simulink model "MatchedFilterFFT_Transpose"  (R2021a)
settings: Solver=FixedStepDiscrete  StartTime=0.0  StopTime=inf  RelTol=1e-3
InitFcn:
  | FFT2D_matrix_init
values from neighbouring files (symbols this model uses):
  columnWindowFun = taylorwin(nCols,10,-40)    [FFT2D_matrix_init.m]
  DTsig_in = numerictype(1,20,18)    [FFT2D_matrix_init.m]
  DTWindowFun = numerictype(1,16+4,13+4)    [FFT2D_matrix_init.m]
  nCols = 64    [FFT2D_matrix_init.m]
  nRows = 256    [FFT2D_matrix_init.m]
  radarDataCube = createRadarDataCubeMod(     txSignalFullPeriod,antennaElement,Fs,Fc,      targetPos, targetVel, targetRCS,      RngMax, RxActiveTime, RngGate,      CPILength, NumCPI, CPILength*pulsePeriod)    [FFT2D_matrix_init.m]
libraries: hdlsllib x35, simulink x13, hwlogicconnlib x2, dsphdlfiltering x1, dsphdlxfrm x1, dspsrcs4 x1
(part 1 of 2)
Description:
  | GenericDesign_AX4Master
  | 
  | Template model for GenericDesign ADC/DAC inports/outports with master/slave DMA connection and AXI4 Master
settings Model: DataTypeOverride=Off  SimulationMode=accelerator  Creator=darenlee  LastModifiedBy=darenlee
settings SolverCC: AlgebraicLoopSolver=TrustRegion
settings DataIOCC: SaveOutput=off  SaveTime=off
settings OptimizationCC: BlockReduction=off  ConditionallyExecuteInputs=off  DefaultParameterBehavior=Inlined
settings DebuggingCC: AlgebraicLoopMsg=error  SingleTaskRateTransMsg=error  SFMachineParentedDataDiag=warning
settings HardwareCC: ProdBitPerPointer=32  ProdBitPerSizeT=32  ProdBitPerPtrDiffT=32  ProdLargestAtomicFloat=None  ProdIntDivRoundTo=Undefined  ProdEndianess=Unspecified  ProdWordSize=32  ProdHWDeviceType=ASIC/FPGA->ASIC/FPGA  TargetBitPerPointer=64  TargetBitPerSizeT=64  TargetBitPerPtrDiffT=64  TargetLongLongMode=on  TargetIntDivRoundTo=Zero  TargetEndianess=LittleEndian  TargetWordSize=64  TargetHWDeviceType=Custom Processor->MATLAB Host Computer  ProdEqTarget=off
settings SFSimCC: CustomCodeUndefinedFunction=UseInterfaceOnly

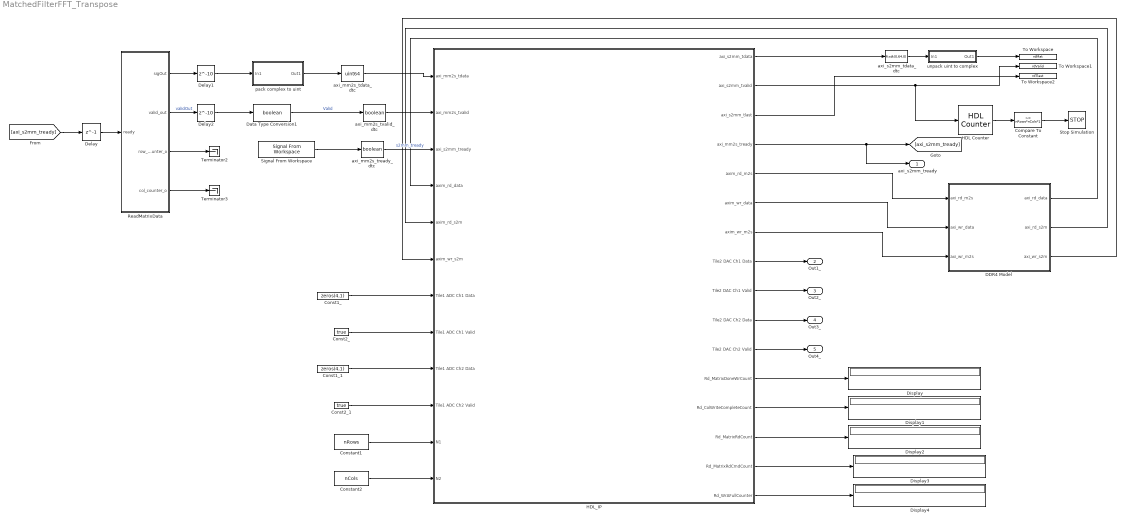
== system MatchedFilterFFT_Transpose ==
  Compare To Constant : simulink/Logic and Bit Operations/Compare To Constant  relop=>=  const=nRows*nCols*1  OutDataTypeStr=boolean
  Const1_ : Constant  Value=zeros(4,1)  OutDataTypeStr=uint64  SampleTime=-1
  Const1_1 : Constant  Value=zeros(4,1)  OutDataTypeStr=uint64  SampleTime=-1
  Const2_ : Constant  Value=true  OutDataTypeStr=boolean  SampleTime=-1
  Const2_1 : Constant  Value=true  OutDataTypeStr=boolean  SampleTime=-1
  Constant1 : Constant  Value=nRows  OutDataTypeStr=uint32  SampleTime=-1
  Constant2 : Constant  Value=nCols  OutDataTypeStr=uint32  SampleTime=-1
  DDR4 Model : Subsystem
  Data Type Conversion1 : DataTypeConversion  OutDataTypeStr=boolean
  Delay : Delay  DelayLength=1
  Delay1 : Delay  DelayLength=10
  Delay2 : Delay  DelayLength=10
  Display{,1..4} (5 alike) : Display
  HDL Counter : hdlsllib/Sources/HDL Counter  CountType=Free running  CountInit=0  CountStep=1  CountMax=25  CountFromType=Initial value  CountFrom=0  CountResetPort=off  CountLoadPort=off  CountEnbPort=on  CountDirPort=off  CountHitOutputPort=off  CountDataType=Unsigned  CountWordLen=32  CountFracLen=0  CountSampTime=1
  HDL_IP : Subsystem  TreatAsAtomicUnit=on
  ReadMatrixData : MATLAB Function  TreatAsAtomicUnit=on  SystemSampleTime=Ts  mask{MatrixInput=radarDataCube, ValidGap=512*3 % 48 clock cycles, Ts=1}
      mask prompts: MatrixInput "Matrix value"; ValidGap "Valid Gap between columns"; Ts "Sample Time"
  Signal From Workspace : dspsrcs4/Signal From Workspace  X=true  Ts=1  nsamps=1  OutputAfterFinalValue=Cyclic repetition  ignoreOrWarnInputAndFrameLengths=off  OutputFrames=off
  Stop Simulation : Stop
  Terminator2 : Terminator
  Terminator3 : Terminator
  To Workspace : ToWorkspace  VariableName=rdMat  SampleTime=-1
      settings: Save2DSignal=2-D array (concatenate along first dimension)
  To Workspace1 : ToWorkspace  VariableName=rdValid  SampleTime=-1
      settings: Save2DSignal=2-D array (concatenate along first dimension)
  To Workspace2 : ToWorkspace  VariableName=rdTlast  SampleTime=-1
      settings: Save2DSignal=2-D array (concatenate along first dimension)
  axi_mm2s_tdata_dtc : DataTypeConversion  OutDataTypeStr=uint64  ConvertRealWorld=Stored Integer (SI)
  axi_mm2s_tready_dtc : DataTypeConversion  OutDataTypeStr=boolean
  axi_mm2s_tvalid_dtc : DataTypeConversion  OutDataTypeStr=boolean
  axi_s2mm_tdata_dtc : DataTypeConversion  OutDataTypeStr=fixdt(0,64,0)  ConvertRealWorld=Stored Integer (SI)
  pack complex to uint : Subsystem
  "unpack uint to complex " : Subsystem
  axi_s2mm_tready : Outport  VectorParamsAs1DForOutWhenUnconnected=off
  Out1_ : Outport  Port=2
  Out2_ : Outport  Port=3
  Out3_ : Outport  Port=4
  Out4_ : Outport  Port=5
  wires:
  HDL_IP/11(Tile2 DAC Ch2 Valid) -> Out4_/1
  axi_mm2s_tvalid_dtc/1 -> HDL_IP/2(axi_mm2s_tvalid)
  Const2_1/1 -> HDL_IP/10(Tile1 ADC Ch2 Valid)
  Const1_1/1 -> HDL_IP/9(Tile1 ADC Ch2 Data)
  HDL_IP/10(Tile2 DAC Ch2 Data) -> Out3_/1
  DDR4 Model/3("axi_wr_s2m ") -> HDL_IP/6(axim_wr_s2m)
  Const2_/1 -> HDL_IP/8(Tile1 ADC Ch1 Valid)
  Const1_/1 -> HDL_IP/7(Tile1 ADC Ch1 Data)
  HDL_IP/9(Tile2 DAC Ch1 Valid) -> Out2_/1
  HDL_IP/8(Tile2 DAC Ch1 Data) -> Out1_/1
  DDR4 Model/1(axi_rd_data) -> HDL_IP/4(axim_rd_data)
  DDR4 Model/2("axi_rd_s2m ") -> HDL_IP/5(axim_rd_s2m)
  HDL_IP/7(axim_wr_m2s) -> DDR4 Model/3(axi_wr_m2s)
  HDL_IP/6(axim_wr_data) -> DDR4 Model/2(axi_wr_data)
  HDL_IP/5(axim_rd_m2s) -> DDR4 Model/1(axi_rd_m2s)
  Signal From Workspace/1 -> axi_mm2s_tready_dtc/1
  Data Type Conversion1/1 -> axi_mm2s_tvalid_dtc/1  "Valid"
  HDL_IP/1(axi_s2mm_tdata) -> axi_s2mm_tdata_dtc/1
  axi_mm2s_tdata_dtc/1 -> HDL_IP/1(axi_mm2s_tdata)
  HDL_IP/4(axi_mm2s_tready) -> axi_s2mm_tready/1, [axi_s2mm_tready]
  axi_mm2s_tready_dtc/1 -> HDL_IP/3(axi_s2mm_tready)  "s2mm_tready"
  ReadMatrixData/4(col_counter_o) -> Terminator3/1
  ReadMatrixData/3(row_counter_o) -> Terminator2/1
  ReadMatrixData/2(valid_out) -> Delay2/1  "validOut"
  ReadMatrixData/1(sigOut) -> Delay1/1
  Compare To Constant/1 -> Stop Simulation/1
  HDL_IP/2(axi_s2mm_tvalid) -> To Workspace1/1, HDL Counter/1
  HDL Counter/1 -> Compare To Constant/1
  axi_s2mm_tdata_dtc/1 -> "unpack uint to complex "/1(In1)
  [axi_s2mm_tready] -> Delay/1
  Delay/1 -> ReadMatrixData/1(ready)
  Constant1/1 -> HDL_IP/11(N1)
  Constant2/1 -> HDL_IP/12(N2)
  Delay2/1 -> Data Type Conversion1/1
  HDL_IP/12(Rd_MatrixDoneWrCount) -> Display/1
  HDL_IP/13(Rd_ColWriteCompleteCount) -> Display1/1
  HDL_IP/14(Rd_MatrixRdCount) -> Display2/1
  HDL_IP/15(Rd_MatrixRdCmdCount) -> Display3/1
  HDL_IP/16(Rd_WrAFullCounter) -> Display4/1
  HDL_IP/3(axi_s2mm_tlast) -> To Workspace2/1
  Delay1/1 -> pack complex to uint/1(In1)
  pack complex to uint/1(Out1) -> axi_mm2s_tdata_dtc/1
  "unpack uint to complex "/1(Out1) -> To Workspace/1

== system MatchedFilterFFT_Transpose/DDR4 Model ==
  axi_rd_m2s : Inport
  axi_wr_data : Inport  Port=2
  axi_wr_m2s : Inport  Port=3
  DDR1 : Subsystem  mask{DDR3_DEPTH=1024, WR_RD_DATAWIDTH=64, INIT_DDR3=off, INIT_ADDR=0, INIT_DATA=fi(zeros(1,1024),0,64,0), OutDataTypeStr=fixdt(0,64,0), READY_DUTY_CYL=1, toggle=off}
      mask prompts: DDR3_DEPTH "DDR DEPTH"; WR_RD_DATAWIDTH "DDR Data Width"; INIT_DDR3 "Initialize DDR"; INIT_ADDR "DDR Initial Address"; INIT_DATA "DDR Initialization data"; OutDataTypeStr "Simulink:blkprm_prompts:UNIFIEDDATATYPE"; READY_DUTY_CYL "READY Duty Cycle"; toggle "Read Valid Toggling"
      mask help: DDR Simulation model
      mask init:
      | if(DDR3_DEPTH<=1)
      |     error('DDR size should be greater than 1' )  
      | end
      | 
      | if(READY_DUTY_CYL>1)
      |   error('should be less than 1' )  
      | end
      |    
      | 
      | %%Initialization Value
      | if(INIT_DDR3==true)
      |     if(isempty(INIT_ADDR))
      |      error('Enter Initial address' )  
      |     end   
      | end
      | 
      | % Check bit-width
      | checkBitdepth = log2(WR_RD_DATAWIDTH);
      | if floor(checkBitdepth) ~= ceil(checkBitdepth)
      |     error('Bit width is not of power base 2!')
      | end
      | 
      | % Check that bit-width matches the initialization data
      | if INIT_DDR3
      |     init_dt_wl = OutDataTypeStr.WordLength;
      |     init_data_wl = INIT_DATA.WordLength;
      |     if init_dt_wl ~= WR_RD_DATAWIDTH
      |         error('Initialization data type and DDR data width should match!')
      |     end
      |     
      |     if init_data_wl ~= WR_RD_DATAWIDTH
      |         error('Initialization data must match DDR data width!')
      |     end    
      | end
      | 
      | 
      | DT_OUTPUT_TYPE = fixdt(0,WR_RD_DATAWIDTH,0);
      mask Help: DDR Simulation model
      mask TypeOptions WR_RD_DATAWIDTH: 32 | 64 | 128
      mask Callback INIT_DDR3:
      | % Get the mask parameter values. This is a cell
      | %   array of character vectors.
      | maskStr = get_param(gcb,'INIT_DDR3');
      | 
      | % The pop-up menu is the first mask parameter.
      | %   Check the value selected in the pop-up
      | if strcmp(maskStr,'on')
      | 
      |     % Set the visibility of both parameters on when
      |     %   User-defined is selected in the pop-up.
      | 
      |     set_param(gcb,'MaskEnables',{'on','on','on','on','on','on','on','on'});
      | 
      | else
      | 
      |     % Turn off the visibility of the Value field
      |     %   when User-defined is not selected.
      | 
      |     set_param(gcb,'MaskEnables',{'on','on','on','off','off','on','on','on'});
      | 
      |     % Set the character vector in the Values field equal to the
      |     % character vector selected in the Gain pop-up menu.
      | 
      |     %maskStr{2}=maskStr{1};
      | 
      | end
      mask TypeOptions OutDataTypeStr: axi_wr_data/OutDataTypeStr | axi_rd_data/OutDataTypeStr
      mask DialogControl DescGroupVar Prompt: DDR
      mask DialogControl DDR3_INIT Prompt: DDR Initialization
      mask DialogControl PARAM_GROUP Prompt: DDR Initialization Parameters
      mask DialogControl OutDataTypeStr Prompt: Data type:
      mask DialogControl READY_DUTY_CYL Tooltip: between 0 to 1
  Terminator : Terminator
  axi_rd_data : Outport
  "axi_rd_s2m " : Outport  Port=2
  "axi_wr_s2m " : Outport  Port=3
  wires:
  axi_rd_m2s/1 -> DDR1/1(axi_rd_m2s)
  axi_wr_data/1 -> DDR1/2(axi_wr_data)
  axi_wr_m2s/1 -> DDR1/3(axi_wr_m2s)
  DDR1/2(axi_rd_data) -> axi_rd_data/1
  DDR1/3(axi_rd_s2m) -> "axi_rd_s2m "/1
  DDR1/4(axi_wr_s2m) -> "axi_wr_s2m "/1
  DDR1/1(load_done) -> Terminator/1

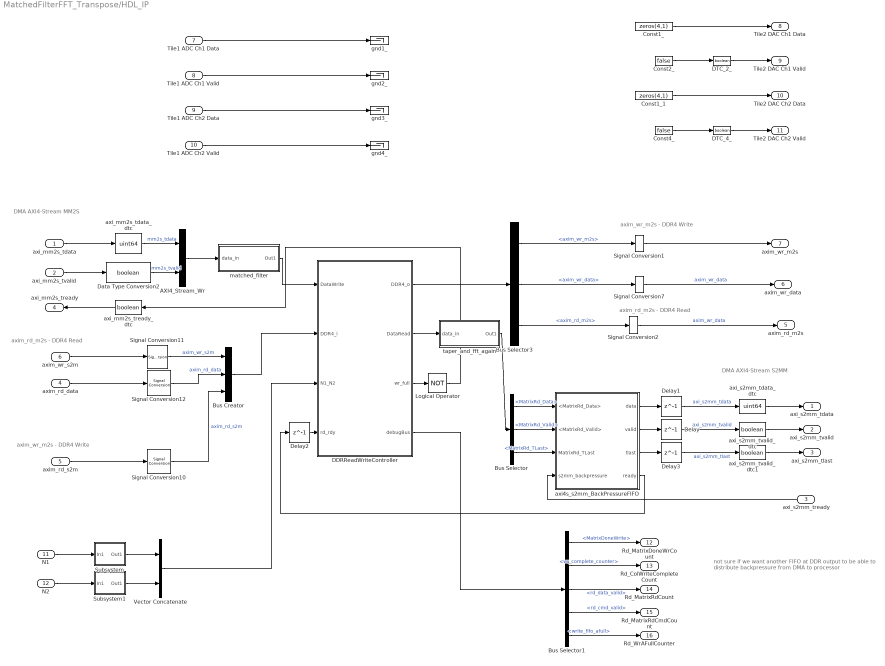
== system MatchedFilterFFT_Transpose/HDL_IP ==
  note: not sure if we want another FIFO at DDR output to be able to distribute backpressure from DMA to processor
  note: DMA AXI4-Stream S2MM
  note: DMA AXI4-Stream MM2S
  note: axim_wr_m2s - DDR4 Write
  note: axim_rd_m2s - DDR4 Read
  note: axim_rd_m2s - DDR4 Read
  note: axim_wr_m2s - DDR4 Write
  axi_mm2s_tdata : Inport
  axi_mm2s_tvalid : Inport  Port=2
  axi_s2mm_tready : Inport  Port=3
  axim_rd_data : Inport  Port=4
  axim_rd_s2m : Inport  Port=5
  axim_wr_s2m : Inport  Port=6
  Tile1 ADC Ch1 Data : Inport  Port=7  OutDataTypeStr=uint64
  Tile1 ADC Ch1 Valid : Inport  Port=8  OutDataTypeStr=boolean
  Tile1 ADC Ch2 Data : Inport  Port=9  OutDataTypeStr=uint64
  Tile1 ADC Ch2 Valid : Inport  Port=10  OutDataTypeStr=boolean
  N1 : Inport  Port=11
  N2 : Inport  Port=12
  AXI4_Stream_Wr : BusCreator  Inputs=2
  Bus Creator : BusCreator  Inputs=3
  Bus Selector : BusSelector  OutputSignals=MatrixRd_Data,MatrixRd_Valid,MatrixRd_TLast
  Bus Selector1 : BusSelector  OutputSignals=MatrixDoneWrite,wr_complete_counter,rd_data_valid,rd_cmd_valid,write_fifo_afull
  Bus Selector3 : BusSelector  OutputSignals=axim_wr_m2s,axim_wr_data,axim_rd_m2s
  Const1_ : Constant  Value=zeros(4,1)  OutDataTypeStr=uint64  SampleTime=-1
  Const1_1 : Constant  Value=zeros(4,1)  OutDataTypeStr=uint64  SampleTime=-1
  Const2_ : Constant  Value=false  OutDataTypeStr=boolean  SampleTime=-1
  Const4_ : Constant  Value=false  OutDataTypeStr=boolean  SampleTime=-1
  DDRReadWriteController : Subsystem
  DTC_2_ : DataTypeConversion  OutDataTypeStr=boolean  ConvertRealWorld=Stored Integer (SI)
  DTC_4_ : DataTypeConversion  OutDataTypeStr=boolean  ConvertRealWorld=Stored Integer (SI)
  Data Type Conversion2 : DataTypeConversion  OutDataTypeStr=boolean
  Delay{,1..3} (4 alike) : Delay  DelayLength=1
  Logical Operator : Logic  Operator=NOT  IconShape=distinctive  AllPortsSameDT=off  OutDataTypeStr=boolean
  Signal Conversion{1..2,7,10..12} (6 alike) : SignalConversion  OverrideOpt=off
  Subsystem : Subsystem  mask{RegVal=uint32(5)}
      mask prompts: RegVal "Default value"
      mask Display: fprintf('Default\n Reg')
  Subsystem1 : Subsystem  mask{RegVal=uint32(5)}
      mask prompts: RegVal "Default value"
      mask Display: fprintf('Default\n Reg')
  Vector Concatenate : Concatenate
  axi4s_s2mm_BackPressureFIFO : Subsystem
  axi_mm2s_tdata_dtc : DataTypeConversion  OutDataTypeStr=uint64  ConvertRealWorld=Stored Integer (SI)
  axi_mm2s_tready_dtc : DataTypeConversion  OutDataTypeStr=boolean
  axi_s2mm_tdata_dtc : DataTypeConversion  OutDataTypeStr=uint64  ConvertRealWorld=Stored Integer (SI)
  axi_s2mm_tvalid_dtc : DataTypeConversion  OutDataTypeStr=boolean
  axi_s2mm_tvalid_dtc1 : DataTypeConversion  OutDataTypeStr=boolean
  gnd1_ : Terminator
  gnd2_ : Terminator
  gnd3_ : Terminator
  gnd4_ : Terminator
  matched_filter : Subsystem
  taper_and_fft_again : Subsystem
  axi_s2mm_tdata : Outport  VectorParamsAs1DForOutWhenUnconnected=off
  axi_s2mm_tvalid : Outport  Port=2  VectorParamsAs1DForOutWhenUnconnected=off
  axi_s2mm_tlast : Outport  Port=3  VectorParamsAs1DForOutWhenUnconnected=off
  axi_mm2s_tready : Outport  Port=4  VectorParamsAs1DForOutWhenUnconnected=off
  axim_rd_m2s : Outport  Port=5  VectorParamsAs1DForOutWhenUnconnected=off
  axim_wr_data : Outport  Port=6  VectorParamsAs1DForOutWhenUnconnected=off
  axim_wr_m2s : Outport  Port=7  VectorParamsAs1DForOutWhenUnconnected=off
  Tile2 DAC Ch1 Data : Outport  Port=8  OutDataTypeStr=uint64
  Tile2 DAC Ch1 Valid : Outport  Port=9  OutDataTypeStr=boolean
  Tile2 DAC Ch2 Data : Outport  Port=10  OutDataTypeStr=uint64
  Tile2 DAC Ch2 Valid : Outport  Port=11  OutDataTypeStr=boolean
  Rd_MatrixDoneWrCount : Outport  Port=12
  Rd_ColWriteCompleteCount : Outport  Port=13
  Rd_MatrixRdCount : Outport  Port=14
  Rd_MatrixRdCmdCount : Outport  Port=15
  Rd_WrAFullCounter : Outport  Port=16
  wires:
  axi_mm2s_tdata/1 -> axi_mm2s_tdata_dtc/1
  DDRReadWriteController/3(wr_full) -> Logical Operator/1
  axi_s2mm_tdata_dtc/1 -> axi_s2mm_tdata/1
  axi_s2mm_tvalid_dtc/1 -> axi_s2mm_tvalid/1
  axi_mm2s_tready_dtc/1 -> axi_mm2s_tready/1
  Signal Conversion10/1 -> Bus Creator/3  "axim_rd_s2m"
  Signal Conversion1/1 -> axim_wr_m2s/1
  axim_rd_data/1 -> Signal Conversion12/1
  Signal Conversion12/1 -> Bus Creator/2  "axim_rd_data"
  axim_rd_s2m/1 -> Signal Conversion10/1
  Signal Conversion7/1 -> axim_wr_data/1  "axim_wr_data"
  axim_wr_s2m/1 -> Signal Conversion11/1
  Tile1 ADC Ch1 Data/1 -> gnd1_/1
  Tile1 ADC Ch1 Valid/1 -> gnd2_/1
  Tile1 ADC Ch2 Data/1 -> gnd3_/1
  Tile1 ADC Ch2 Valid/1 -> gnd4_/1
  Const1_/1 -> Tile2 DAC Ch1 Data/1
  Const2_/1 -> DTC_2_/1
  DTC_2_/1 -> Tile2 DAC Ch1 Valid/1
  Const1_1/1 -> Tile2 DAC Ch2 Data/1
  Const4_/1 -> DTC_4_/1
  DTC_4_/1 -> Tile2 DAC Ch2 Valid/1
  Signal Conversion11/1 -> Bus Creator/1  "axim_wr_s2m"
  Signal Conversion2/1 -> axim_rd_m2s/1  "axim_wr_data"
  axi_mm2s_tdata_dtc/1 -> AXI4_Stream_Wr/1  "mm2s_tdata"
  axi_mm2s_tvalid/1 -> Data Type Conversion2/1
  Data Type Conversion2/1 -> AXI4_Stream_Wr/2  "mm2s_tvalid"
  Bus Selector3/1 -> Signal Conversion1/1  "<axim_wr_m2s>"
  Bus Selector3/2 -> Signal Conversion7/1  "<axim_wr_data>"
  Bus Selector3/3 -> Signal Conversion2/1  "<axim_rd_m2s>"
  AXI4_Stream_Wr/1 -> matched_filter/1(data_in)
  Bus Creator/1 -> DDRReadWriteController/2(DDR4_i)
  DDRReadWriteController/1(DDR4_o) -> Bus Selector3/1
  Delay1/1 -> axi_s2mm_tdata_dtc/1  "axi_s2mm_tdata"
  Bus Selector/1 -> axi4s_s2mm_BackPressureFIFO/1(<MatrixRd_Data>)  "<MatrixRd_Data>"
  Bus Selector/2 -> axi4s_s2mm_BackPressureFIFO/2(<MatrixRd_Valid>)  "<MatrixRd_Valid>"
  axi_s2mm_tready/1 -> axi4s_s2mm_BackPressureFIFO/4(s2mm_backpressure)
  axi4s_s2mm_BackPressureFIFO/1(data) -> Delay1/1
  axi4s_s2mm_BackPressureFIFO/2(valid) -> Delay/1
  Delay/1 -> axi_s2mm_tvalid_dtc/1  "axi_s2mm_tvalid"
  axi4s_s2mm_BackPressureFIFO/4(ready) -> Delay2/1
  Delay2/1 -> DDRReadWriteController/4(rd_rdy)
  Logical Operator/1 -> axi_mm2s_tready_dtc/1
  N2/1 -> Subsystem1/1(In1)
  Vector Concatenate/1 -> DDRReadWriteController/3(N1_N2)
  N1/1 -> Subsystem/1(In1)
  Subsystem/1(Out1) -> Vector Concatenate/1
  Subsystem1/1(Out1) -> Vector Concatenate/2
  DDRReadWriteController/4(debugBus) -> Bus Selector1/1
  Bus Selector1/1 -> Rd_MatrixDoneWrCount/1  "<MatrixDoneWrite>"
  Bus Selector1/2 -> Rd_ColWriteCompleteCount/1  "<wr_complete_counter>"
  Bus Selector1/3 -> Rd_MatrixRdCount/1  "<rd_data_valid>"
  Bus Selector1/4 -> Rd_MatrixRdCmdCount/1  "<rd_cmd_valid>"
  Bus Selector1/5 -> Rd_WrAFullCounter/1  "<write_fifo_afull>"
  Bus Selector/3 -> axi4s_s2mm_BackPressureFIFO/3(MatrixRd_TLast)  "<MatrixRd_TLast>"
  axi4s_s2mm_BackPressureFIFO/3(tlast) -> Delay3/1
  Delay3/1 -> axi_s2mm_tvalid_dtc1/1  "axi_s2mm_tlast"
  axi_s2mm_tvalid_dtc1/1 -> axi_s2mm_tlast/1
  matched_filter/1(Out1) -> DDRReadWriteController/1(DataWrite)
  DDRReadWriteController/2(DataRead) -> taper_and_fft_again/1(data_in)
  taper_and_fft_again/1(Out1) -> Bus Selector/1

== system MatchedFilterFFT_Transpose/pack complex to uint ==
  In1 : Inport
  Bit Concat : hdlsllib/Logic and Bit Operations/Bit Concat  numInputs=2
  Complex to Real-Imag : ComplexToRealImag
  Data Type Conversion2 : DataTypeConversion  OutDataTypeStr=DTsig_in
  Out1 : Outport
  wires:
  Complex to Real-Imag/2 -> Bit Concat/2
  Data Type Conversion2/1 -> Complex to Real-Imag/1  "Data"
  Complex to Real-Imag/1 -> Bit Concat/1
  Bit Concat/1 -> Out1/1
  In1/1 -> Data Type Conversion2/1

== system MatchedFilterFFT_Transpose/unpack uint to complex  ==
  In1 : Inport
  Bit Slice : hdlsllib/Logic and Bit Operations/Bit Slice  lidx=63  ridx=32
      settings: SourceProductBaseCode=SL
  Bit Slice1 : hdlsllib/Logic and Bit Operations/Bit Slice  lidx=31  ridx=0
      settings: SourceProductBaseCode=SL
  Data Type Conversion : DataTypeConversion  OutDataTypeStr=fixdt(1,32,22)  ConvertRealWorld=Stored Integer (SI)
  Real-Imag to Complex : RealImagToComplex
  Out1 : Outport
  wires:
  Bit Slice1/1 -> Real-Imag to Complex/2
  Bit Slice/1 -> Real-Imag to Complex/1
  Data Type Conversion/1 -> Out1/1
  Real-Imag to Complex/1 -> Data Type Conversion/1
  In1/1 -> Bit Slice1/1, Bit Slice/1

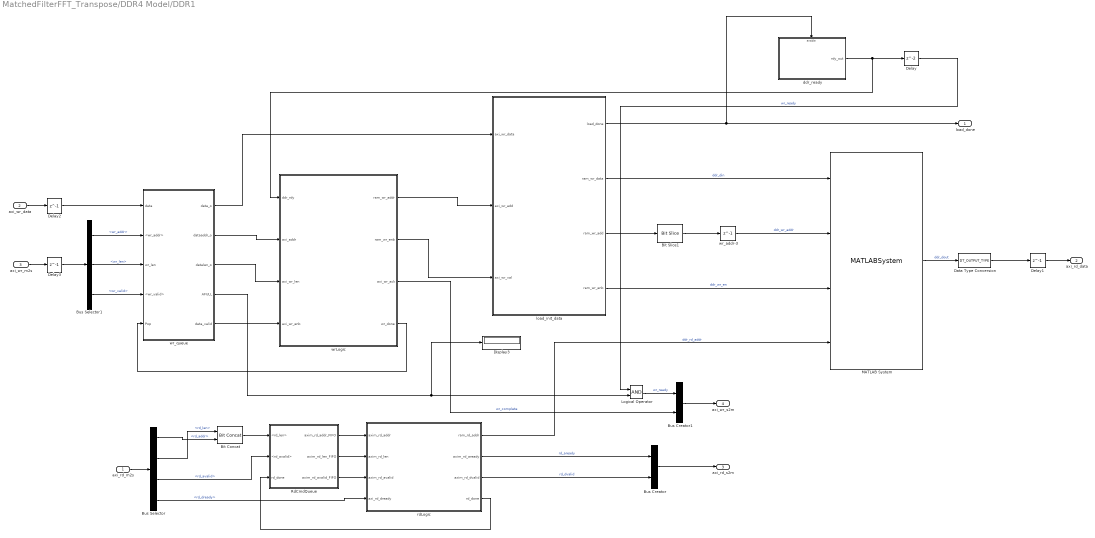
== system MatchedFilterFFT_Transpose/DDR4 Model/DDR1 ==
  axi_rd_m2s : Inport
  axi_wr_data : Inport  Port=2  OutDataTypeStr=fixdt(0,64,0)
  axi_wr_m2s : Inport  Port=3
  Bit Concat : hdlsllib/Logic and Bit Operations/Bit Concat  numInputs=2
  Bit Slice1 : hdlsllib/Logic and Bit Operations/Bit Slice  lidx=15  ridx=0
      settings: SourceProductBaseCode=SL
  Bus Creator : BusCreator  Inputs=2
  Bus Creator1 : BusCreator  Inputs=2
  Bus Selector : BusSelector  OutputSignals=rd_addr,rd_len,rd_avalid,rd_dready
  Bus Selector1 : BusSelector  OutputSignals=wr_addr,wr_len,wr_valid
  Data Type Conversion : DataTypeConversion  OutDataTypeStr=DT_OUTPUT_TYPE
  Delay : Delay
  Delay1 : Delay  DelayLength=1
  Delay2 : Delay  DelayLength=1
  Delay3 : Delay  DelayLength=1
  Display3 : Display
  Logical Operator : Logic  AllPortsSameDT=off  OutDataTypeStr=boolean
  MATLAB System : MATLABSystem  System=hdl.RAM  RAMType=Simple dual port  WriteOutputValue=New data  RAMInitialValue=0  SimulateUsing=Code generation
      mask Type: hdl.RAM
      mask Display:
      | disp(['Simple' char(10) 'Dual Port' char(10) 'RAM']);
      | port_label('input',1,'din');
      | port_label('input',2,'wr_addr');
      | port_label('input',3,'wr_en');
      | port_label('input',4,'rd_addr');
      | port_label('output',1,'rd_dout');
  RdCmdQueue : Subsystem
  ddr_ready : Subsystem
  load_init_data : MATLAB Function  TreatAsAtomicUnit=on
  rdLogic : Subsystem
  wrLogic : Subsystem
  wr_addr-3 : Delay  DelayLength=1
  wr_queue : Subsystem
  load_done : Outport  VectorParamsAs1DForOutWhenUnconnected=off
  axi_rd_data : Outport  Port=2  OutDataTypeStr=fixdt(0,64,0)  VectorParamsAs1DForOutWhenUnconnected=off
  axi_rd_s2m : Outport  Port=3  VectorParamsAs1DForOutWhenUnconnected=off
  axi_wr_s2m : Outport  Port=4  VectorParamsAs1DForOutWhenUnconnected=off
  wires:
  RdCmdQueue/1(axim_rd_addr_FIFO) -> rdLogic/1(axim_rd_addr)
  Bit Concat/1 -> RdCmdQueue/1(<rd_len>)
  rdLogic/4(rd_done) -> RdCmdQueue/3(rd_done)
  RdCmdQueue/3(axim_rd_avalid_FIFO) -> rdLogic/3(axim_rd_avalid)
  RdCmdQueue/2(axim_rd_len_FIFO) -> rdLogic/2(axim_rd_len)
  Bus Selector/3 -> RdCmdQueue/2(<rd_avalid>)  "<rd_avalid>"
  Bus Selector/2 -> Bit Concat/1  "<rd_len>"
  Data Type Conversion/1 -> Delay1/1
  Delay3/1 -> Bus Selector1/1
  Delay2/1 -> wr_queue/1(data)
  axi_wr_data/1 -> Delay2/1
  load_init_data/2(ram_wr_data) -> MATLAB System/1  "ddr_din"
  Delay/1 -> Logical Operator/1  "wr_ready"
  wrLogic/3(axi_wr_ack) -> Bus Creator1/2  "wr_complete"
  Bus Creator1/1 -> axi_wr_s2m/1
  ddr_ready/1(rdy_out) -> wrLogic/1(ddr_rdy), Delay/1
  rdLogic/3(axim_rd_dvalid) -> Bus Creator/2  "rd_dvalid"
  Bus Creator/1 -> axi_rd_s2m/1
  rdLogic/2(axim_rd_aready) -> Bus Creator/1  "rd_aready"
  Bus Selector1/2 -> wr_queue/3(wr_len)  "<wr_len>"
  Bus Selector1/3 -> wr_queue/4(<wr_valid>)  "<wr_valid>"
  axi_wr_m2s/1 -> Delay3/1
  axi_rd_m2s/1 -> Bus Selector/1
  Bus Selector/4 -> rdLogic/4(axi_rd_dready)  "<rd_dready>"
  Bus Selector/1 -> Bit Concat/2  "<rd_addr>"
  wr_addr-3/1 -> MATLAB System/2  "ddr_wr_addr"
  wrLogic/2(ram_wr_enb) -> load_init_data/3(axi_wr_val)
  wrLogic/1(ram_wr_addr) -> load_init_data/2(axi_wr_add)
  rdLogic/1(ram_rd_addr) -> MATLAB System/4  "ddr_rd_addr"
  MATLAB System/1 -> Data Type Conversion/1  "ddr_dout"
  load_init_data/1(load_done) -> load_done/1, ddr_ready/Enable
  load_init_data/3(ram_wr_add) -> Bit Slice1/1
  load_init_data/4(ram_wr_enb) -> MATLAB System/3  "ddr_wr_en"
  Delay1/1 -> axi_rd_data/1
  Bit Slice1/1 -> wr_addr-3/1
  Bus Selector1/1 -> wr_queue/2(<wr_addr>)  "<wr_addr>"
  wrLogic/4(wr_done) -> wr_queue/5(Pop)
  Logical Operator/1 -> Bus Creator1/1  "wr_ready"
  wr_queue/4(AFULL) -> Display3/1, Logical Operator/2
  wr_queue/2(dataaddr_o) -> wrLogic/2(axi_addr)
  wr_queue/1(data_o) -> load_init_data/1(axi_wr_data)
  wr_queue/3(datalen_o) -> wrLogic/3(axi_wr_len)
  wr_queue/5(data_valid) -> wrLogic/4(axi_wr_enb)

== system MatchedFilterFFT_Transpose/HDL_IP/DDRReadWriteController ==
  DataWrite : Inport
  DDR4_i : Inport  Port=2
  N1_N2 : Inport  Port=3
  rd_rdy : Inport  Port=4
  Bus Creator1 : BusCreator  Inputs=3
  Bus Selector1 : BusSelector  OutputSignals=mm2s_tdata,mm2s_tvalid
  Bus Selector2 : BusSelector  OutputSignals=axim_wr_s2m,axim_rd_data,axim_rd_s2m
  Data Type Conversion1 : DataTypeConversion  OutDataTypeStr=uint64  ConvertRealWorld=Stored Integer (SI)
  TransposeMatrix : Subsystem  TreatAsAtomicUnit=on
  DDR4_o : Outport
  DataRead : Outport  Port=2
  wr_full : Outport  Port=3
  debugBus : Outport  Port=4
  wires:
  TransposeMatrix/1(TRWr_m2s) -> Bus Creator1/1  "axim_wr_m2s"
  Bus Selector2/3 -> TransposeMatrix/5(rd_s2m)  "<axim_rd_s2m>"
  Data Type Conversion1/1 -> Bus Creator1/2  "axim_wr_data"
  DDR4_i/1 -> Bus Selector2/1
  TransposeMatrix/3(rd_m2s) -> Bus Creator1/3  "axim_rd_m2s"
  Bus Creator1/1 -> DDR4_o/1
  Bus Selector2/1 -> TransposeMatrix/3(Wr_s2m)  "<axim_wr_s2m>"
  TransposeMatrix/2(TRWr_data) -> Data Type Conversion1/1
  TransposeMatrix/4(matrix_rd_out) -> DataRead/1
  Bus Selector2/2 -> TransposeMatrix/4(rd_data)  "<axim_rd_data>"
  Bus Selector1/2 -> TransposeMatrix/2(ValidIn)  "<mm2s_tvalid>"
  Bus Selector1/1 -> TransposeMatrix/1(DataIn)  "<mm2s_tdata>"
  DataWrite/1 -> Bus Selector1/1
  TransposeMatrix/5(wr_full) -> wr_full/1
  rd_rdy/1 -> TransposeMatrix/6(rd_rdy)
  N1_N2/1 -> TransposeMatrix/7(N1_N2)
  TransposeMatrix/6(debugBus) -> debugBus/1

== system MatchedFilterFFT_Transpose/HDL_IP/Subsystem ==
  In1 : Inport
  Constant : Constant  Value=RegVal  SampleTime=-1
  Data Type Duplicate : DataTypeDuplicate
  Delay3 : Delay  DelayLength=1
  Switch : Switch  Criteria=u2 ~= 0
  Out1 : Outport
  wires:
  Delay3/1 -> Out1/1
  In1/1 -> Data Type Duplicate/1, Switch/1, Switch/2
  Switch/1 -> Delay3/1
  Constant/1 -> Switch/3, Data Type Duplicate/2

== system MatchedFilterFFT_Transpose/HDL_IP/Subsystem1 ==
  In1 : Inport
  Constant : Constant  Value=RegVal  SampleTime=-1
  Data Type Duplicate : DataTypeDuplicate
  Delay3 : Delay  DelayLength=1
  Switch : Switch  Criteria=u2 ~= 0
  Out1 : Outport
  wires:
  Delay3/1 -> Out1/1
  In1/1 -> Data Type Duplicate/1, Switch/1, Switch/2
  Switch/1 -> Delay3/1
  Constant/1 -> Switch/3, Data Type Duplicate/2

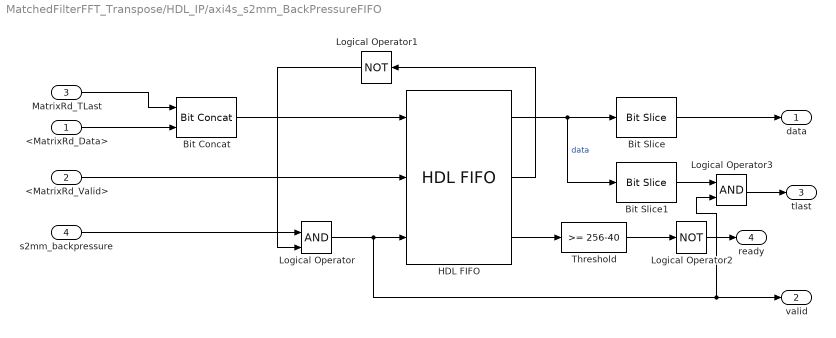
== system MatchedFilterFFT_Transpose/HDL_IP/axi4s_s2mm_BackPressureFIFO ==
  <MatrixRd_Data> : Inport
  <MatrixRd_Valid> : Inport  Port=2
  MatrixRd_TLast : Inport  Port=3
  s2mm_backpressure : Inport  Port=4
  Bit Concat : hdlsllib/Logic and Bit Operations/Bit Concat  numInputs=2
  Bit Slice : hdlsllib/Logic and Bit Operations/Bit Slice  lidx=63  ridx=0
      settings: SourceProductBaseCode=SL
  Bit Slice1 : hdlsllib/Logic and Bit Operations/Bit Slice  lidx=64  ridx=64
      settings: SourceProductBaseCode=SL
  HDL FIFO : hdlsllib/HDL RAMs/HDL FIFO  fifo_size=256  mode=FWFT  ratio=1  push_msg=Warning  pop_msg=Warning  show_empty=on  show_full=off  show_num=on  LabelModeActiveChoice_Mode=FWFT
      settings: SourceProductBaseCode=SL
  Logical Operator : Logic  IconShape=distinctive  AllPortsSameDT=off  OutDataTypeStr=boolean
  Logical Operator1 : Logic  Operator=NOT  IconShape=distinctive  AllPortsSameDT=off  OutDataTypeStr=boolean
  Logical Operator2 : Logic  Operator=NOT  IconShape=distinctive  AllPortsSameDT=off  OutDataTypeStr=boolean
  Logical Operator3 : Logic  AllPortsSameDT=off  OutDataTypeStr=boolean
  Threshold : simulink/Logic and Bit Operations/Compare To Constant  relop=>=  const=256-40  OutDataTypeStr=boolean
  data : Outport
  valid : Outport  Port=2
  tlast : Outport  Port=3
  ready : Outport  Port=4
  wires:
  <MatrixRd_Valid>/1 -> HDL FIFO/2
  <MatrixRd_Data>/1 -> Bit Concat/2
  Logical Operator1/1 -> Logical Operator/2
  HDL FIFO/2 -> Logical Operator1/1
  HDL FIFO/3 -> Threshold/1
  Logical Operator/1 -> HDL FIFO/3, Logical Operator3/2, valid/1
  HDL FIFO/1 -> Bit Slice1/1, Bit Slice/1  "data"
  s2mm_backpressure/1 -> Logical Operator/1
  Threshold/1 -> Logical Operator2/1
  Logical Operator2/1 -> ready/1
  Bit Concat/1 -> HDL FIFO/1
  MatrixRd_TLast/1 -> Bit Concat/1
  Bit Slice/1 -> data/1
  Bit Slice1/1 -> Logical Operator3/1
  Logical Operator3/1 -> tlast/1

== system MatchedFilterFFT_Transpose/HDL_IP/matched_filter ==
  note: lose some bits for now. pack into a fixdt(1,32,25)
  data_in : Inport
  AXI4_Stream_Wr : BusCreator  Inputs=2
  Bus Selector1 : BusSelector  OutputSignals=mm2s_tdata,mm2s_tvalid
  Data Type Conversion : DataTypeConversion  OutDataTypeStr=fixdt(1,32,24)
  Discrete FIR Filter HDL Optimized : dsphdlfiltering/Discrete FIR Filter HDL Optimized  NumeratorSource=Property  Numerator=matchingCoeff.'  NumeratorPrototype=[]  FilterStructure=Direct form systolic  SerializationOption=Minimum number of cycles between valid input samples  NumberOfCycles=2  NumberOfMultipliers=2  SimulateUsing=Code generation  roundingMode=Floor  overflowMode=off  CoefficientsDataTypeStr=Inherit: Same word length as input  CoefficientsMin=[]  CoefficientsMax=[]  OutputMin=[]  OutputMax=[]  ResetInputPort=off  HDLGlobalReset=off
      settings: SourceProductBaseCode=DS
  Terminator : Terminator
  line_start_marker : Subsystem
  pack complex to uint64 : Subsystem
  "unpack uint to DTsig_in " : Subsystem
  Out1 : Outport
  wires:
  data_in/1 -> Bus Selector1/1
  Bus Selector1/1 -> "unpack uint to DTsig_in "/1(In1)  "<mm2s_tdata>"
  AXI4_Stream_Wr/1 -> Out1/1
  "unpack uint to DTsig_in "/1(Out1) -> Discrete FIR Filter HDL Optimized/1  "input_matrix"
  Bus Selector1/2 -> line_start_marker/1(<mm2s_tvalid>), Discrete FIR Filter HDL Optimized/2  "<mm2s_tvalid>"
  Data Type Conversion/1 -> pack complex to uint64/1(In1)  "fft1_out"
  pack complex to uint64/1(Out1) -> AXI4_Stream_Wr/1  "mm2s_tdata"
  line_start_marker/1(Out1) -> Terminator/1  "line_start_marker"
  Discrete FIR Filter HDL Optimized/1 -> Data Type Conversion/1
  Discrete FIR Filter HDL Optimized/2 -> AXI4_Stream_Wr/2  "mm2s_tvalid"

== system MatchedFilterFFT_Transpose/HDL_IP/taper_and_fft_again ==
  note: match FFT delay
  data_in : Inport
  Bus Creator : BusCreator  Inputs=3
  Bus Selector1 : BusSelector  OutputSignals=MatrixRd_Data,MatrixRd_Valid,MatrixRd_TLast
  Data Type Conversion : DataTypeConversion  OutDataTypeStr=fixdt(1,32,21)
  Delay : Delay  DelayLength=173
  FFT HDL Optimized : dsphdlxfrm/FFT HDL Optimized  FFTLength=nCols  Architecture=Streaming Radix 2^2  ComplexMultiplication=Use 4 multipliers and 2 adders  BitReversedOutput=off  BitReversedInput=off  Normalize=on  SimulateUsing=Code generation  RoundingMethod=Floor  ResetInputPort=off  StartOutputPort=off  EndOutputPort=off
      settings: SourceProductBaseCode=DS
  Signal Copy : SignalConversion  OverrideOpt=off
  Subsystem Reference : Subsystem  ReferencedSubsystem=window_taper  windowFun=fi(columnWindowFun,DTWindowFun)
  line_start_marker : Subsystem
  pack complex to uint64 : Subsystem
  "unpack uint64 to complex " : Subsystem
  Out1 : Outport
  wires:
  data_in/1 -> Bus Selector1/1
  Bus Selector1/1 -> "unpack uint64 to complex "/1(In1)  "<MatrixRd_Data>"
  Bus Selector1/2 -> line_start_marker/1(<mm2s_tvalid>), Signal Copy/1  "<MatrixRd_Valid>"
  "unpack uint64 to complex "/1(data_in) -> Subsystem Reference/1  "input_matrix_2"
  line_start_marker/1(Out1) -> Subsystem Reference/3  "line_start_marker_2"
  FFT HDL Optimized/1 -> Data Type Conversion/1
  FFT HDL Optimized/2 -> Bus Creator/2  "MatrixRd_Valid"
  Data Type Conversion/1 -> pack complex to uint64/1(In1)  "fft2_out"
  Bus Selector1/3 -> Delay/1  "<MatrixRd_TLast>"
  Delay/1 -> Bus Creator/3  "MatrixRd_TLast"
  pack complex to uint64/1(Out1) -> Bus Creator/1  "MatrixRd_Data"
  Bus Creator/1 -> Out1/1
  Signal Copy/1 -> Subsystem Reference/2  "input_valid_2"
  Subsystem Reference/2 -> FFT HDL Optimized/2
  Subsystem Reference/1 -> FFT HDL Optimized/1

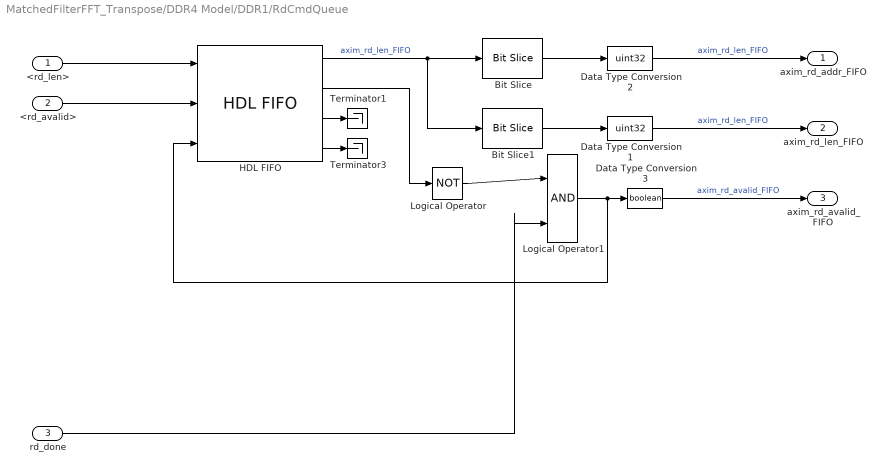
== system MatchedFilterFFT_Transpose/DDR4 Model/DDR1/RdCmdQueue ==
  <rd_len> : Inport
  <rd_avalid> : Inport  Port=2
  rd_done : Inport  Port=3
  Bit Slice : hdlsllib/Logic and Bit Operations/Bit Slice  lidx=31  ridx=0
      settings: SourceProductBaseCode=SL
  Bit Slice1 : hdlsllib/Logic and Bit Operations/Bit Slice  lidx=63  ridx=32
      settings: SourceProductBaseCode=SL
  Data Type Conversion1 : DataTypeConversion  OutDataTypeStr=uint32
  Data Type Conversion2 : DataTypeConversion  OutDataTypeStr=uint32
  Data Type Conversion3 : DataTypeConversion  OutDataTypeStr=boolean
  HDL FIFO : hdlsllib/HDL RAMs/HDL FIFO  fifo_size=1024  mode=FWFT  ratio=1  push_msg=Warning  pop_msg=Warning  show_empty=on  show_full=on  show_num=on  LabelModeActiveChoice_Mode=FWFT
      settings: SourceProductBaseCode=SL
  Logical Operator : Logic  Operator=NOT  IconShape=distinctive  AllPortsSameDT=off  OutDataTypeStr=boolean
  Logical Operator1 : Logic  IconShape=distinctive  AllPortsSameDT=off  OutDataTypeStr=boolean
  Terminator1 : Terminator
  Terminator3 : Terminator
  axim_rd_addr_FIFO : Outport  VectorParamsAs1DForOutWhenUnconnected=off
  axim_rd_len_FIFO : Outport  Port=2
  axim_rd_avalid_FIFO : Outport  Port=3
  wires:
  Data Type Conversion2/1 -> axim_rd_addr_FIFO/1  "axim_rd_len_FIFO"
  Bit Slice/1 -> Data Type Conversion2/1
  Bit Slice1/1 -> Data Type Conversion1/1
  Data Type Conversion1/1 -> axim_rd_len_FIFO/1  "axim_rd_len_FIFO"
  rd_done/1 -> Logical Operator1/2
  <rd_len>/1 -> HDL FIFO/1
  HDL FIFO/1 -> Bit Slice1/1, Bit Slice/1  "axim_rd_len_FIFO"
  Data Type Conversion3/1 -> axim_rd_avalid_FIFO/1  "axim_rd_avalid_FIFO"
  Logical Operator/1 -> Logical Operator1/1
  <rd_avalid>/1 -> HDL FIFO/2
  HDL FIFO/2 -> Logical Operator/1
  Logical Operator1/1 -> Data Type Conversion3/1, HDL FIFO/3
  HDL FIFO/3 -> Terminator1/1
  HDL FIFO/4 -> Terminator3/1

== system MatchedFilterFFT_Transpose/DDR4 Model/DDR1/ddr_ready ==
  Enable : EnablePort
  Data Type Conversion : DataTypeConversion  OutDataTypeStr=boolean
  Pulse Generator : DiscretePulseGenerator  Period=1000  PulseWidth=1000 * READY_DUTY_CYL  SampleTime=-1
  rdy_out : Outport  VectorParamsAs1DForOutWhenUnconnected=off
  wires:
  Data Type Conversion/1 -> rdy_out/1
  Pulse Generator/1 -> Data Type Conversion/1

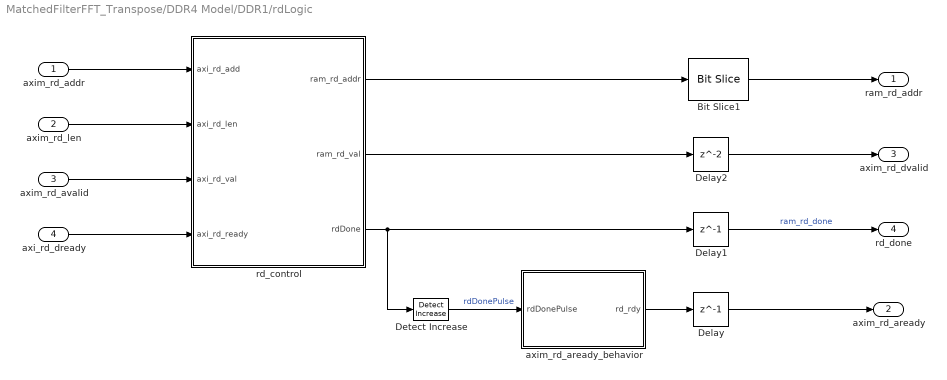
== system MatchedFilterFFT_Transpose/DDR4 Model/DDR1/rdLogic ==
  axim_rd_addr : Inport
  axim_rd_len : Inport  Port=2
  axim_rd_avalid : Inport  Port=3
  axi_rd_dready : Inport  Port=4
  Bit Slice1 : hdlsllib/Logic and Bit Operations/Bit Slice  lidx=15  ridx=0
      settings: SourceProductBaseCode=SL
  Delay : Delay  DelayLength=1
  Delay1 : Delay  DelayLength=1
  Delay2 : Delay
  Detect Increase : simulink/Logic and Bit Operations/Detect Increase  vinit=0.0  OutDataTypeStr=boolean
  axim_rd_aready_behavior : MATLAB Function  TreatAsAtomicUnit=on
  rd_control : MATLAB Function  TreatAsAtomicUnit=on
  ram_rd_addr : Outport  VectorParamsAs1DForOutWhenUnconnected=off
  axim_rd_aready : Outport  Port=2  VectorParamsAs1DForOutWhenUnconnected=off
  axim_rd_dvalid : Outport  Port=3  VectorParamsAs1DForOutWhenUnconnected=off
  rd_done : Outport  Port=4  VectorParamsAs1DForOutWhenUnconnected=off
  wires:
  Delay1/1 -> rd_done/1  "ram_rd_done"
  rd_control/2(ram_rd_val) -> Delay2/1
  axim_rd_len/1 -> rd_control/2(axi_rd_len)
  Delay2/1 -> axim_rd_dvalid/1
  axi_rd_dready/1 -> rd_control/4(axi_rd_ready)
  Bit Slice1/1 -> ram_rd_addr/1
  axim_rd_avalid/1 -> rd_control/3(axi_rd_val)
  rd_control/1(ram_rd_addr) -> Bit Slice1/1
  axim_rd_addr/1 -> rd_control/1(axi_rd_add)
  axim_rd_aready_behavior/1(rd_rdy) -> Delay/1
  rd_control/3(rdDone) -> Detect Increase/1, Delay1/1
  Detect Increase/1 -> axim_rd_aready_behavior/1(rdDonePulse)  "rdDonePulse"
  Delay/1 -> axim_rd_aready/1

== system MatchedFilterFFT_Transpose/DDR4 Model/DDR1/wrLogic ==
  ddr_rdy : Inport
  axi_addr : Inport  Port=2
  axi_wr_len : Inport  Port=3
  axi_wr_enb : Inport  Port=4
  Add : Sum  AccumDataTypeStr=uint32
  Bit Shift : hdlsllib/Logic and Bit Operations/Bit Shift  mode=Shift Right Arithmetic  N=log2(WR_RD_DATAWIDTH/8)
  Logical Operator : Logic  Operator=OR  IconShape=distinctive  AllPortsSameDT=off  OutDataTypeStr=boolean
  Wr_control : Subsystem
  ddr_ack_d1 : Delay  DelayLength=1
  ddr_reday_d1 : Delay  DelayLength=1
  ddr_reday_d6 : Delay  DelayLength=4
  ram_wr_addr : Outport  VectorParamsAs1DForOutWhenUnconnected=off
  ram_wr_enb : Outport  Port=2  VectorParamsAs1DForOutWhenUnconnected=off
  axi_wr_ack : Outport  Port=3  VectorParamsAs1DForOutWhenUnconnected=off
  wr_done : Outport  Port=4
  wires:
  Bit Shift/1 -> Add/1
  Logical Operator/1 -> Wr_control/1(ddr_wr_rdy)
  ddr_reday_d1/1 -> Logical Operator/1
  axi_addr/1 -> Bit Shift/1
  ddr_ack_d1/1 -> axi_wr_ack/1
  ddr_reday_d6/1 -> Logical Operator/2, ddr_reday_d1/1
  Wr_control/3(ram_addr) -> Add/2
  Add/1 -> ram_wr_addr/1
  Wr_control/2(axim_ack) -> ddr_ack_d1/1
  axi_wr_enb/1 -> Wr_control/2(wr_enb)
  ddr_rdy/1 -> ddr_reday_d6/1
  axi_wr_len/1 -> Wr_control/3(wr_len)
  Wr_control/1(valAddEnb) -> ram_wr_enb/1
  Wr_control/4(wr_done) -> wr_done/1

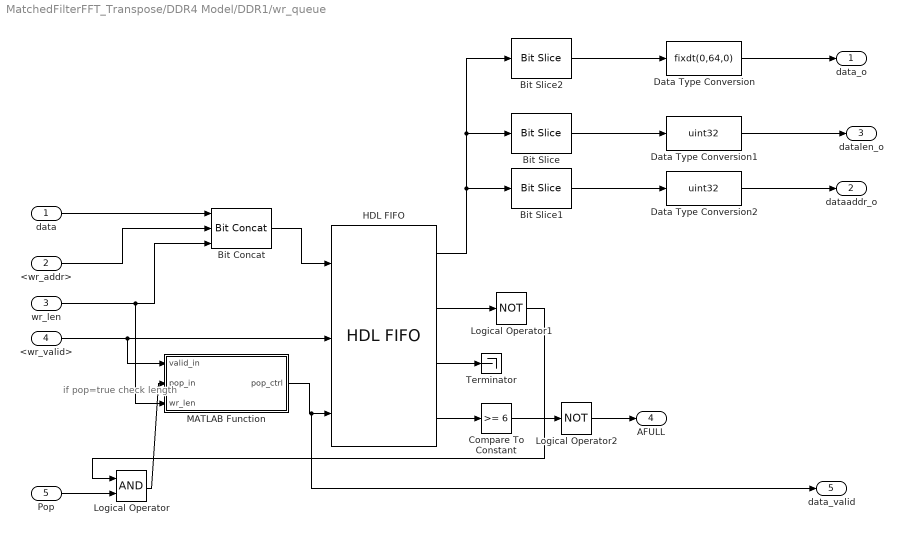
== system MatchedFilterFFT_Transpose/DDR4 Model/DDR1/wr_queue ==
  note: if pop=true
      | check length
  data : Inport
  <wr_addr> : Inport  Port=2
  wr_len : Inport  Port=3
  <wr_valid> : Inport  Port=4
  Pop : Inport  Port=5
  Bit Concat : hdlsllib/Logic and Bit Operations/Bit Concat  numInputs=3
  Bit Slice : hdlsllib/Logic and Bit Operations/Bit Slice  lidx=31  ridx=0
      settings: SourceProductBaseCode=SL
  Bit Slice1 : hdlsllib/Logic and Bit Operations/Bit Slice  lidx=63  ridx=32
      settings: SourceProductBaseCode=SL
  Bit Slice2 : hdlsllib/Logic and Bit Operations/Bit Slice  lidx=127  ridx=64
      settings: SourceProductBaseCode=SL
  Compare To Constant : simulink/Logic and Bit Operations/Compare To Constant  relop=>=  const=6  OutDataTypeStr=boolean
  Data Type Conversion : DataTypeConversion  OutDataTypeStr=fixdt(0,64,0)  ConvertRealWorld=Stored Integer (SI)
  Data Type Conversion1 : DataTypeConversion  OutDataTypeStr=uint32  ConvertRealWorld=Stored Integer (SI)
  Data Type Conversion2 : DataTypeConversion  OutDataTypeStr=uint32  ConvertRealWorld=Stored Integer (SI)
  HDL FIFO : hdlsllib/HDL RAMs/HDL FIFO  fifo_size=8  mode=FWFT  ratio=1  push_msg=Warning  pop_msg=Warning  show_empty=on  show_full=on  show_num=on  LabelModeActiveChoice_Mode=FWFT
      settings: SourceProductBaseCode=SL
  Logical Operator : Logic  AllPortsSameDT=off  OutDataTypeStr=boolean
  Logical Operator1 : Logic  Operator=NOT  AllPortsSameDT=off  OutDataTypeStr=boolean
  Logical Operator2 : Logic  Operator=NOT  AllPortsSameDT=off  OutDataTypeStr=boolean
  MATLAB Function : MATLAB Function  TreatAsAtomicUnit=on
  Terminator : Terminator
  data_o : Outport
  dataaddr_o : Outport  Port=2
  datalen_o : Outport  Port=3
  AFULL : Outport  Port=4
  data_valid : Outport  Port=5
  wires:
  Data Type Conversion1/1 -> datalen_o/1
  Logical Operator1/1 -> Logical Operator/1
  Pop/1 -> Logical Operator/2
  <wr_valid>/1 -> MATLAB Function/1(valid_in), HDL FIFO/2
  HDL FIFO/2 -> Logical Operator1/1
  data/1 -> Bit Concat/1
  <wr_addr>/1 -> Bit Concat/2
  wr_len/1 -> MATLAB Function/3(wr_len), Bit Concat/3
  Bit Concat/1 -> HDL FIFO/1
  HDL FIFO/1 -> Bit Slice2/1, Bit Slice/1, Bit Slice1/1
  Bit Slice2/1 -> Data Type Conversion/1
  Bit Slice/1 -> Data Type Conversion1/1
  Data Type Conversion/1 -> data_o/1
  Bit Slice1/1 -> Data Type Conversion2/1
  Data Type Conversion2/1 -> dataaddr_o/1
  HDL FIFO/3 -> Terminator/1
  HDL FIFO/4 -> Compare To Constant/1
  Compare To Constant/1 -> Logical Operator2/1
  Logical Operator2/1 -> AFULL/1
  Logical Operator/1 -> MATLAB Function/2(pop_in)
  MATLAB Function/1(pop_ctrl) -> data_valid/1, HDL FIFO/3

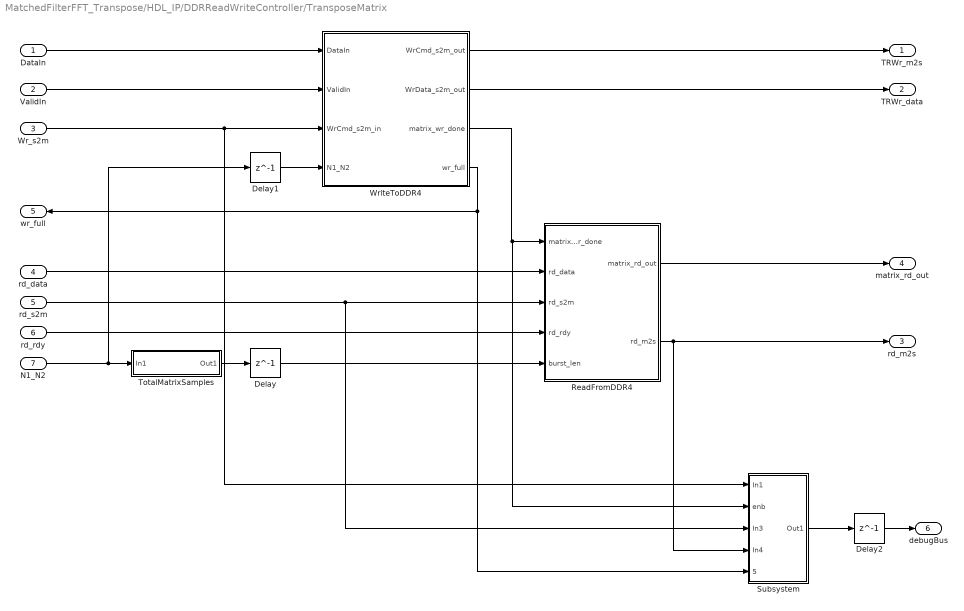
== system MatchedFilterFFT_Transpose/HDL_IP/DDRReadWriteController/TransposeMatrix ==
  DataIn : Inport
  ValidIn : Inport  Port=2
  Wr_s2m : Inport  Port=3  SampleTime=1
  rd_data : Inport  Port=4  SampleTime=1
  rd_s2m : Inport  Port=5  SampleTime=1
  rd_rdy : Inport  Port=6
  N1_N2 : Inport  Port=7
  Delay : Delay  DelayLength=1
  Delay1 : Delay  DelayLength=1
  Delay2 : Delay  DelayLength=1
  ReadFromDDR4 : Subsystem
  Subsystem : Subsystem
  TotalMatrixSamples : Subsystem
  WriteToDDR4 : Subsystem
  TRWr_m2s : Outport  SampleTime=1  VectorParamsAs1DForOutWhenUnconnected=off
  TRWr_data : Outport  Port=2  SampleTime=1  VectorParamsAs1DForOutWhenUnconnected=off
  rd_m2s : Outport  Port=3
  matrix_rd_out : Outport  Port=4
  wr_full : Outport  Port=5
  debugBus : Outport  Port=6
  wires:
  DataIn/1 -> WriteToDDR4/1(DataIn)
  ValidIn/1 -> WriteToDDR4/2(ValidIn)
  Wr_s2m/1 -> Subsystem/1(In1), WriteToDDR4/3(WrCmd_s2m_in)
  WriteToDDR4/1(WrCmd_s2m_out) -> TRWr_m2s/1
  WriteToDDR4/2(WrData_s2m_out) -> TRWr_data/1
  rd_data/1 -> ReadFromDDR4/2(rd_data)
  rd_s2m/1 -> Subsystem/3(In3), ReadFromDDR4/3(rd_s2m)
  ReadFromDDR4/2(rd_m2s) -> rd_m2s/1, Subsystem/4(In4)
  WriteToDDR4/3(matrix_wr_done) -> Subsystem/2(enb), ReadFromDDR4/1(matrix_wr_done)
  ReadFromDDR4/1(matrix_rd_out) -> matrix_rd_out/1
  WriteToDDR4/4(wr_full) -> wr_full/1, Subsystem/5(mm2s_backpressure)
  rd_rdy/1 -> ReadFromDDR4/4(rd_rdy)
  N1_N2/1 -> Delay1/1, TotalMatrixSamples/1(In1)
  TotalMatrixSamples/1(Out1) -> Delay/1
  Delay/1 -> ReadFromDDR4/5(burst_len)
  Delay1/1 -> WriteToDDR4/4(N1_N2)
  Delay2/1 -> debugBus/1
  Subsystem/1(Out1) -> Delay2/1

== system MatchedFilterFFT_Transpose/HDL_IP/matched_filter/line_start_marker ==
  <mm2s_tvalid> : Inport
  AND : Logic  IconShape=distinctive  AllPortsSameDT=off  OutDataTypeStr=boolean
  Compare To Constant : simulink/Logic and Bit Operations/Compare To Constant  relop===  const=0  OutDataTypeStr=boolean
  HDL Counter : hdlsllib/Sources/HDL Counter  CountType=Count limited  CountInit=0  CountStep=1  CountMax=nRows-1  CountFromType=Initial value  CountFrom=0  CountResetPort=off  CountLoadPort=off  CountEnbPort=on  CountDirPort=off  CountHitOutputPort=off  CountDataType=Unsigned  CountWordLen=16  CountFracLen=0  CountSampTime=1
  Out1 : Outport
  wires:
  <mm2s_tvalid>/1 -> AND/1, HDL Counter/1
  HDL Counter/1 -> Compare To Constant/1
  Compare To Constant/1 -> AND/2
  AND/1 -> Out1/1

== system MatchedFilterFFT_Transpose/HDL_IP/matched_filter/pack complex to uint64 ==
  In1 : Inport
  Bit Concat : hdlsllib/Logic and Bit Operations/Bit Concat  numInputs=2
  Complex to Real-Imag : ComplexToRealImag
  Out1 : Outport
  wires:
  Complex to Real-Imag/2 -> Bit Concat/2
  In1/1 -> Complex to Real-Imag/1  "Data"
  Complex to Real-Imag/1 -> Bit Concat/1
  Bit Concat/1 -> Out1/1

== system MatchedFilterFFT_Transpose/HDL_IP/matched_filter/unpack uint to DTsig_in  ==
  In1 : Inport
  Bit Slice : hdlsllib/Logic and Bit Operations/Bit Slice  lidx=DTsig_in.WordLength*2 -1  ridx=DTsig_in.WordLength
      settings: SourceProductBaseCode=SL
  Bit Slice1 : hdlsllib/Logic and Bit Operations/Bit Slice  lidx=DTsig_in.WordLength - 1  ridx=0
      settings: SourceProductBaseCode=SL
  Data Type Conversion : DataTypeConversion  OutDataTypeStr=DTsig_in  ConvertRealWorld=Stored Integer (SI)
  Real-Imag to Complex : RealImagToComplex
  Out1 : Outport
  wires:
  Bit Slice1/1 -> Real-Imag to Complex/2
  Bit Slice/1 -> Real-Imag to Complex/1
  Data Type Conversion/1 -> Out1/1
  Real-Imag to Complex/1 -> Data Type Conversion/1
  In1/1 -> Bit Slice1/1, Bit Slice/1

== system MatchedFilterFFT_Transpose/HDL_IP/taper_and_fft_again/line_start_marker ==
  <mm2s_tvalid> : Inport
  AND : Logic  IconShape=distinctive  AllPortsSameDT=off  OutDataTypeStr=boolean
  Compare To Constant : simulink/Logic and Bit Operations/Compare To Constant  relop===  const=0  OutDataTypeStr=boolean
  HDL Counter : hdlsllib/Sources/HDL Counter  CountType=Count limited  CountInit=0  CountStep=1  CountMax=nCols-1  CountFromType=Initial value  CountFrom=0  CountResetPort=off  CountLoadPort=off  CountEnbPort=on  CountDirPort=off  CountHitOutputPort=off  CountDataType=Unsigned  CountWordLen=16  CountFracLen=0  CountSampTime=1
  Out1 : Outport
  wires:
  <mm2s_tvalid>/1 -> AND/1, HDL Counter/1
  HDL Counter/1 -> Compare To Constant/1
  Compare To Constant/1 -> AND/2
  AND/1 -> Out1/1

== system MatchedFilterFFT_Transpose/HDL_IP/taper_and_fft_again/pack complex to uint64 ==
  In1 : Inport
  Bit Concat : hdlsllib/Logic and Bit Operations/Bit Concat  numInputs=2
  Complex to Real-Imag : ComplexToRealImag
  Out1 : Outport
  wires:
  Complex to Real-Imag/2 -> Bit Concat/2
  In1/1 -> Complex to Real-Imag/1  "Data"
  Complex to Real-Imag/1 -> Bit Concat/1
  Bit Concat/1 -> Out1/1

== system MatchedFilterFFT_Transpose/HDL_IP/taper_and_fft_again/unpack uint64 to complex  ==
  In1 : Inport
  Bit Slice : hdlsllib/Logic and Bit Operations/Bit Slice  lidx=63  ridx=32
      settings: SourceProductBaseCode=SL
  Bit Slice1 : hdlsllib/Logic and Bit Operations/Bit Slice  lidx=31  ridx=0
      settings: SourceProductBaseCode=SL
  Data Type Conversion : DataTypeConversion  OutDataTypeStr=fixdt(1,32,24)  ConvertRealWorld=Stored Integer (SI)
  Real-Imag to Complex : RealImagToComplex
  data_in : Outport
  wires:
  Bit Slice1/1 -> Real-Imag to Complex/2
  Bit Slice/1 -> Real-Imag to Complex/1
  Data Type Conversion/1 -> data_in/1
  Real-Imag to Complex/1 -> Data Type Conversion/1
  In1/1 -> Bit Slice1/1, Bit Slice/1

== system MatchedFilterFFT_Transpose/DDR4 Model/DDR1/wrLogic/Wr_control ==
  ddr_wr_rdy : Inport
  wr_enb : Inport  Port=2
  wr_len : Inport  Port=3
  AckGen : Subsystem
  Delay : Delay  DelayLength=1
  MATLAB Function : MATLAB Function  TreatAsAtomicUnit=on
  Unit Delay : UnitDelay  SampleTime=-1  HasFrameUpgradeWarning=on
  valAddEnb : Outport  VectorParamsAs1DForOutWhenUnconnected=off
  axim_ack : Outport  Port=2  VectorParamsAs1DForOutWhenUnconnected=off
  ram_addr : Outport  Port=3  VectorParamsAs1DForOutWhenUnconnected=off
  wr_done : Outport  Port=4
  wires:
  ddr_wr_rdy/1 -> AckGen/3(ddr_wr_rdy)
  AckGen/3(ram_addr) -> ram_addr/1
  Unit Delay/1 -> MATLAB Function/3(wr_ack), axim_ack/1
  MATLAB Function/1(wr_leng) -> AckGen/1(axiWrLen)
  AckGen/1(ack) -> Unit Delay/1
  wr_len/1 -> MATLAB Function/2(axi_wr_length)
  AckGen/2(ValAddEnb) -> valAddEnb/1
  wr_enb/1 -> MATLAB Function/1(axi_wr_en), AckGen/2(wrEnb)
  MATLAB Function/2(wr_done_o) -> Delay/1
  Delay/1 -> wr_done/1

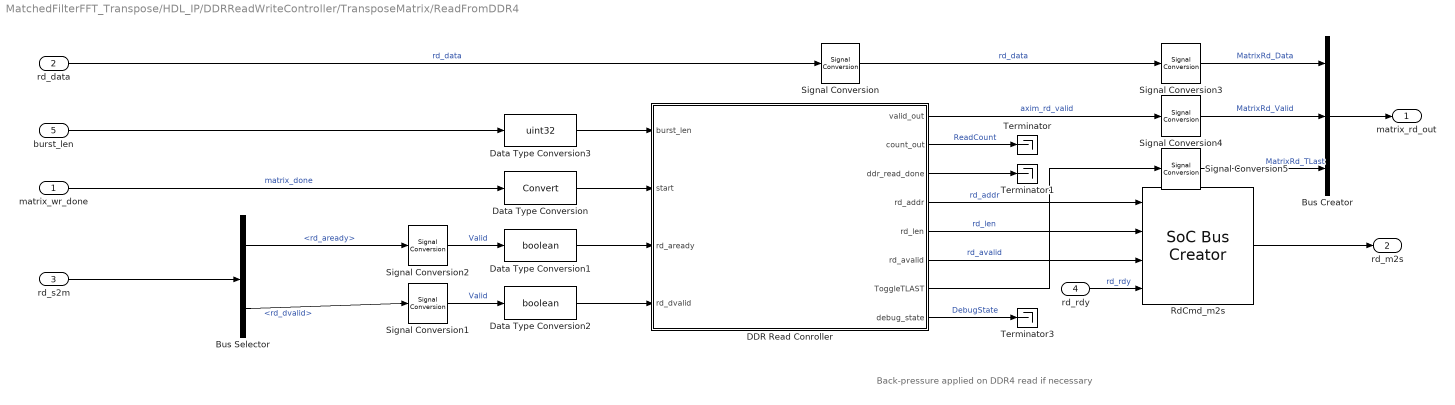
== system MatchedFilterFFT_Transpose/HDL_IP/DDRReadWriteController/TransposeMatrix/ReadFromDDR4 ==
  note: Back-pressure applied on DDR4 read if necessary
  matrix_wr_done : Inport
  rd_data : Inport  Port=2
  rd_s2m : Inport  Port=3
  rd_rdy : Inport  Port=4
  burst_len : Inport  Port=5
  Bus Creator : BusCreator  Inputs=3
  Bus Selector : BusSelector  OutputSignals=rd_aready,rd_dvalid
  DDR Read Conroller : MATLAB Function  TreatAsAtomicUnit=on
  Data Type Conversion : DataTypeConversion
  Data Type Conversion1 : DataTypeConversion  OutDataTypeStr=boolean
  Data Type Conversion2 : DataTypeConversion  OutDataTypeStr=boolean
  Data Type Conversion3 : DataTypeConversion  OutDataTypeStr=uint32
  RdCmd_m2s : hwlogicconnlib/SoC Bus Creator  Protocol=Random access read  ctrltype=Ready
      settings: SourceProductBaseCode=HW
  Signal Conversion{,1..5} (6 alike) : SignalConversion  OverrideOpt=off
  Terminator : Terminator
  Terminator1 : Terminator
  Terminator3 : Terminator
  matrix_rd_out : Outport
  rd_m2s : Outport  Port=2
  wires:
  Signal Conversion1/1 -> Data Type Conversion2/1  "Valid"
  Signal Conversion/1 -> Signal Conversion3/1  "rd_data"
  RdCmd_m2s/1 -> rd_m2s/1
  rd_data/1 -> Signal Conversion/1  "rd_data"
  rd_s2m/1 -> Bus Selector/1
  matrix_wr_done/1 -> Data Type Conversion/1  "matrix_done"
  burst_len/1 -> Data Type Conversion3/1
  Signal Conversion2/1 -> Data Type Conversion1/1  "Valid"
  DDR Read Conroller/2(count_out) -> Terminator/1  "ReadCount"
  DDR Read Conroller/1(valid_out) -> Signal Conversion4/1  "axim_rd_valid"
  DDR Read Conroller/3(ddr_read_done) -> Terminator1/1
  rd_rdy/1 -> RdCmd_m2s/4  "rd_rdy"
  DDR Read Conroller/7(ToggleTLAST) -> Signal Conversion5/1
  DDR Read Conroller/8(debug_state) -> Terminator3/1  "DebugState"
  Signal Conversion3/1 -> Bus Creator/1  "MatrixRd_Data"
  Signal Conversion4/1 -> Bus Creator/2  "MatrixRd_Valid"
  Bus Creator/1 -> matrix_rd_out/1
  Bus Selector/1 -> Signal Conversion2/1  "<rd_aready>"
  Bus Selector/2 -> Signal Conversion1/1  "<rd_dvalid>"
  Data Type Conversion/1 -> DDR Read Conroller/2(start)
  Data Type Conversion1/1 -> DDR Read Conroller/3(rd_aready)
  Data Type Conversion2/1 -> DDR Read Conroller/4(rd_dvalid)
  DDR Read Conroller/6(rd_avalid) -> RdCmd_m2s/3  "rd_avalid"
  DDR Read Conroller/4(rd_addr) -> RdCmd_m2s/1  "rd_addr"
  DDR Read Conroller/5(rd_len) -> RdCmd_m2s/2  "rd_len"
  Data Type Conversion3/1 -> DDR Read Conroller/1(burst_len)
  Signal Conversion5/1 -> Bus Creator/3  "MatrixRd_TLast"

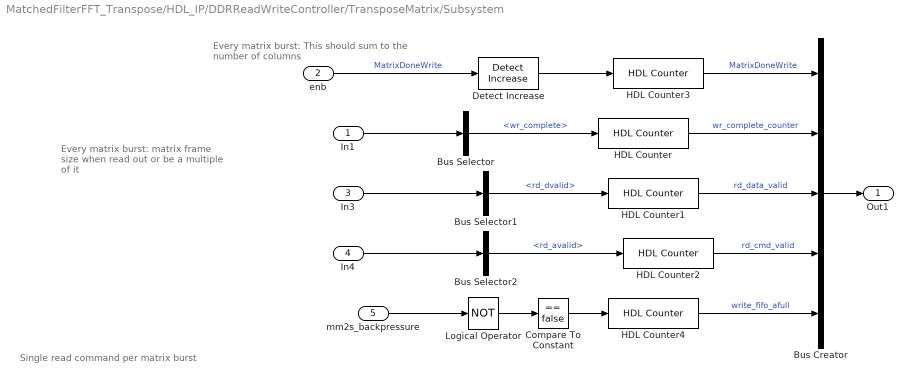
== system MatchedFilterFFT_Transpose/HDL_IP/DDRReadWriteController/TransposeMatrix/Subsystem ==
  note: Single read command per matrix burst
  note: Every matrix burst:
      |  matrix frame size when read out
      | or be a multiple of it
  note: Every matrix burst:
      | This should sum to the number of columns
  In1 : Inport
  enb : Inport  Port=2
  In3 : Inport  Port=3
  In4 : Inport  Port=4
  mm2s_backpressure : Inport  Port=5
  Bus Creator : BusCreator  Inputs=5
  Bus Selector : BusSelector  OutputSignals=wr_complete
  Bus Selector1 : BusSelector  OutputSignals=rd_dvalid
  Bus Selector2 : BusSelector  OutputSignals=rd_avalid
  Compare To Constant : simulink/Logic and Bit Operations/Compare To Constant  relop===  const=false  OutDataTypeStr=boolean
  Detect Increase : simulink/Logic and Bit Operations/Detect Increase  vinit=0.0  OutDataTypeStr=boolean
  HDL Counter{,1..4} (5 alike) : hdlsllib/Sources/HDL Counter  CountType=Free running  CountInit=0  CountStep=1  CountMax=25  CountFromType=Initial value  CountFrom=0  CountResetPort=off  CountLoadPort=off  CountEnbPort=on  CountDirPort=off  CountHitOutputPort=off  CountDataType=Unsigned  CountWordLen=32  CountFracLen=0  CountSampTime=1
  Logical Operator : Logic  Operator=NOT  IconShape=distinctive  AllPortsSameDT=off  OutDataTypeStr=boolean
  Out1 : Outport
  wires:
  HDL Counter/1 -> Bus Creator/2  "wr_complete_counter"
  In3/1 -> Bus Selector1/1
  Bus Selector2/1 -> HDL Counter2/1  "<rd_avalid>"
  HDL Counter2/1 -> Bus Creator/4  "rd_cmd_valid"
  enb/1 -> Detect Increase/1  "MatrixDoneWrite"
  HDL Counter1/1 -> Bus Creator/3  "rd_data_valid"
  In1/1 -> Bus Selector/1
  In4/1 -> Bus Selector2/1
  Bus Creator/1 -> Out1/1
  Bus Selector/1 -> HDL Counter/1  "<wr_complete>"
  Bus Selector1/1 -> HDL Counter1/1  "<rd_dvalid>"
  HDL Counter3/1 -> Bus Creator/1  "MatrixDoneWrite"
  mm2s_backpressure/1 -> Logical Operator/1
  Logical Operator/1 -> Compare To Constant/1
  HDL Counter4/1 -> Bus Creator/5  "write_fifo_afull"
  Compare To Constant/1 -> HDL Counter4/1
  Detect Increase/1 -> HDL Counter3/1
